simulink model "ejemplo_H"  (R2024b)
settings: Solver=VariableStepAuto  StartTime=0.0  StopTime=5  RelTol=1e-3
undefined symbols (not defined in the file): A, B, C, K
settings Model: Creator=juanm  LastModifiedBy=juanm

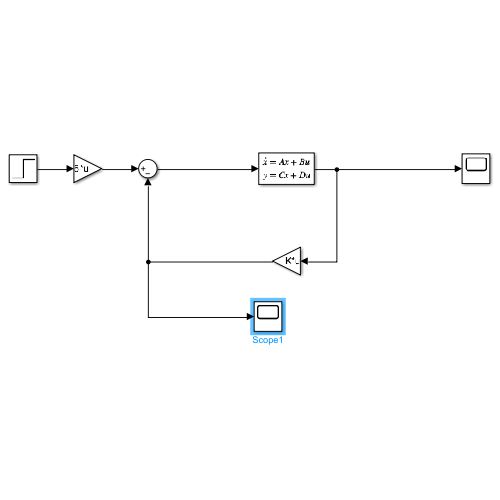
[thumbnail: Simulink's stored preview of the top-level diagram]
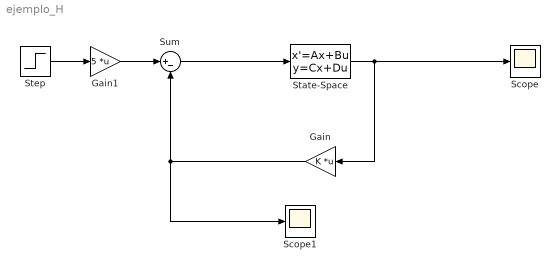
== system ejemplo_H ==
  Gain : Gain  Gain=K  Multiplication=Matrix(K*u)
  Gain1 : Gain  Gain=5  Multiplication=Matrix(K*u)
  Scope : Scope
  Scope1 : Scope
  State-Space : StateSpace  A=A  B=B  C=C  D=[0;0]  InitialCondition=[0;0]
  Step : Step  Time=5  After=5  SampleTime=0
  Sum : Sum  Inputs=|+-
  wires:
  Sum/1 -> State-Space/1
  State-Space/1 -> Gain/1, Scope/1
  Gain/1 -> Sum/2, Scope1/1
  Step/1 -> Gain1/1
  Gain1/1 -> Sum/1
